simulink library "components"  (R2024b)
settings: Solver=VariableStepAuto  StartTime=0.0  StopTime=10.0  RelTol=1e-3
undefined symbols (not defined in the file): dt
settings Model: Creator=rayen  LastModifiedBy=rayen

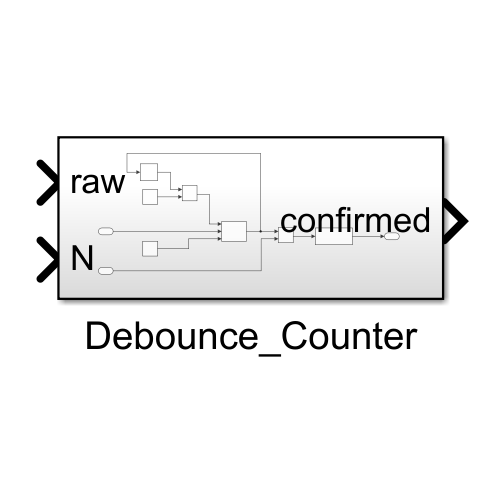
[thumbnail: Simulink's stored preview of the top-level diagram]
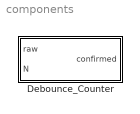
== system components ==
  Debounce_Counter : Subsystem

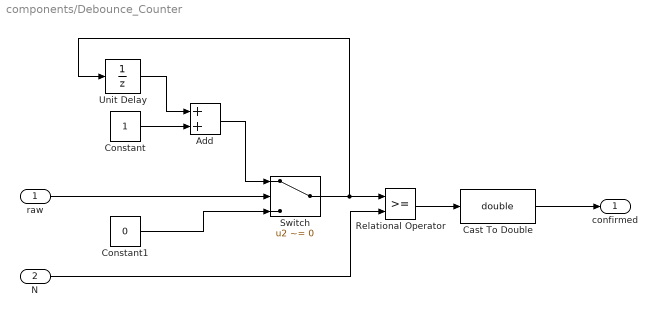
== system components/Debounce_Counter ==
  raw : Inport
  N : Inport  Port=2
  Add : Sum
  Cast To Double : DataTypeConversion  OutDataTypeStr=double  SaturateOnIntegerOverflow=off  RndMeth=Floor
  Constant : Constant
  Constant1 : Constant  Value=0
  Relational Operator : RelationalOperator  OutDataTypeStr=boolean  RndMeth=Simplest  InputSameDT=off
  Switch : Switch  Criteria=u2 ~= 0  SaturateOnIntegerOverflow=off  InputSameDT=off
  Unit Delay : UnitDelay  SampleTime=dt  HasFrameUpgradeWarning=on
  confirmed : Outport
  wires:
  Unit Delay/1 -> Add/1
  Constant/1 -> Add/2
  Add/1 -> Switch/1
  raw/1 -> Switch/2
  Constant1/1 -> Switch/3
  Switch/1 -> Relational Operator/1, Unit Delay/1
  N/1 -> Relational Operator/2
  Relational Operator/1 -> Cast To Double/1
  Cast To Double/1 -> confirmed/1
